simulink model "M1DCSSimulator_M1BcoordinateSystem"  (R2021a)
settings: Solver=VariableStepAuto  StartTime=0.0  StopTime=10.0  RelTol=1e-3
undefined symbols (not defined in the file or in its folder): DiscIntNeverNeededParam
settings Model: Creator=tranka  LastModifiedBy=tranka

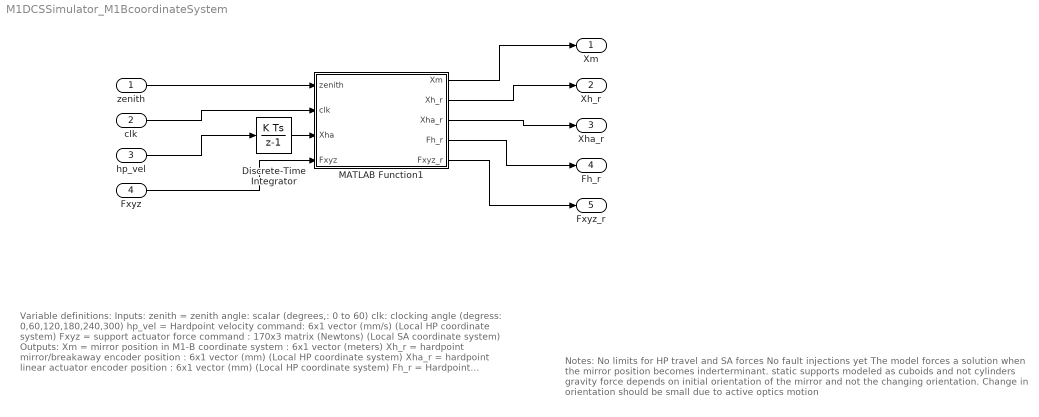
== system M1DCSSimulator_M1BcoordinateSystem ==
  note: Variable definitions:
      |
      | Inputs:
      | zenith = zenith angle: scalar (degrees,: 0 to 60)
      | clk: clocking angle (degress: 0,60,120,180,240,300)
      | hp_vel = Hardpoint velocity command: 6x1 vector (mm/s) (Local HP coordinate system)
      | Fxyz = support actuator force command : 170x3 matrix (Newtons) (Local SA coordinate system)
      |
      | Outputs:
      | Xm = mirror position in M1-B coordinate system : 6x1 vector (meters)
      | Xh_r = hardpoint mirror/breakaway encoder position : 6x1 vector (mm) (Local HP coordinate system)
      | Xha_r = hardpoint linear actuator encoder position : 6x1 vector (mm) (Local HP coordinate system)
      | Fh_r = Hardpoint loadcell readout : 6x1 vector (Newtons) (Local HP coordinate system)
      | FXYZ_r = support actuator force readback : 165x3 matrix (M1B coordinate system. Need to be fixed to local SA coordinate system)
  note: Notes:
      | No limits for HP travel and SA forces
      | No fault injections yet
      | The model forces a solution when the mirror position becomes inderterminant.
      | static supports modeled as cuboids and not cylinders
      | gravity force depends on initial orientation of the mirror and not the changing orientation.
      | Change in orientation should be small due to active optics motion
  zenith : Inport
  clk : Inport  Port=2
  hp_vel : Inport  Port=3
  Fxyz : Inport  Port=4
  Discrete-Time Integrator : DiscreteIntegrator  SampleTime=-1  ICPrevOutput=DiscIntNeverNeededParam  ICPrevScaledInput=DiscIntNeverNeededParam
  MATLAB Function1 : MATLAB Function  TreatAsAtomicUnit=on
  Xm : Outport
  Xh_r : Outport  Port=2
  Xha_r : Outport  Port=3
  Fh_r : Outport  Port=4
  Fxyz_r : Outport  Port=5
  wires:
  Discrete-Time Integrator/1 -> MATLAB Function1/3(Xha)
  zenith/1 -> MATLAB Function1/1(zenith)
  clk/1 -> MATLAB Function1/2(clk)
  hp_vel/1 -> Discrete-Time Integrator/1
  Fxyz/1 -> MATLAB Function1/4(Fxyz)
  MATLAB Function1/1(Xm) -> Xm/1
  MATLAB Function1/2(Xh_r) -> Xh_r/1
  MATLAB Function1/3(Xha_r) -> Xha_r/1
  MATLAB Function1/4(Fh_r) -> Fh_r/1
  MATLAB Function1/5(Fxyz_r) -> Fxyz_r/1

== matlab function M1DCSSimulator_M1BcoordinateSystem/MATLAB Function1 ==
  data: zenith input; clk input; Xm output; Xha input; Fxyz input; Xh_r output; Xha_r output; Fh_r output; Fxyz_r output
function [Xm,Xh_r,Xha_r,Fh_r, Fxyz_r] = mirror(zenith,clk, Xha,Fxyz)
%% fix input coordinates, indexes, units etc
% pass the support actuator to output
% In future implement SA force limits or disable a few actuators.
Fxyz_r = Fxyz;
sign_matrix = [-1    -1    -1
    -1    -1    -1
    -1    -1    -1
    -1    -1    -1
     1     1    -1
     1     1    -1
    -1    -1    -1
    -1    -1    -1
    -1    -1    -1
    -1    -1    -1
    -1    -1    -1
     1     1    -1
    -1    -1    -1
    -1    -1    -1
    -1    -1    -1
    -1    -1    -1
     1     1    -1
     1     1    -1
    -1    -1    -1
    -1    -1    -1
    -1    -1    -1
    -1    -1    -1
     1     1    -1
     1     1    -1
    -1    -1    -1
    -1    -1    -1
    -1    -1    -1
     1     1    -1
     1     1    -1
    -1    -1    -1
    -1    -1    -1
     1     1    -1
     1     1    -1
     1     1    -1
     1     1    -1
     1     1    -1
     1     1    -1
     1     1    -1
     1     1    -1
     1     1    -1
     1     1    -1
     1     1    -1
     1     1    -1
     1     1    -1
     1     1    -1
     1     1    -1
     1     1    -1
     1     1    -1
     1     1    -1
     1     1    -1
     1     1    -1
     1     1    -1
     1     1    -1
     1     1    -1
     1     1    -1
     1     1    -1
     1     1    -1
     1     1    -1
     1     1    -1
     1     1    -1
     1     1    -1
     1     1    -1
     1     1    -1
     1     1    -1
     1     1    -1
     1     1    -1
     1     1    -1
     1     1    -1
     1     1    -1
     1     1    -1
     1     1    -1
     1     1    -1
     1     1    -1
     1     1    -1
     1     1    -1
     1     1    -1
     1     1    -1
     1     1    -1
     1     1    -1
     1     1    -1
     1     1    -1
     1     1    -1
     1     1    -1
     1     1    -1
     1     1    -1
     1     1    -1
     1     1    -1
     1     1    -1
     1     1    -1
     1     1    -1
     1     1    -1
     1     1    -1
     1     1    -1
     1     1    -1
     1     1    -1
     1     1    -1
     1     1    -1
     1     1    -1
     1     1    -1
     1     1    -1
     1     1    -1
     1     1    -1
     1     1    -1
     1     1    -1
     1     1    -1
     1     1    -1
     1     1    -1
     1     1    -1
     1     1    -1
     1     1    -1
     1     1    -1
     1     1    -1
     1     1    -1
     1     1    -1
     1     1    -1
     1     1    -1
     1     1    -1
    -1    -1    -1
    -1    -1    -1
    -1    -1    -1
    -1    -1    -1
    -1    -1    -1
     1     1    -1
    -1    -1    -1
    -1    -1    -1
    -1    -1    -1
    -1    -1    -1
     1     1    -1
     1     1    -1
    -1    -1    -1
    -1    -1    -1
    -1    -1    -1
    -1    -1    -1
     1     1    -1
     1     1    -1
    -1    -1    -1
    -1    -1    -1
    -1    -1    -1
     1     1    -1
     1     1    -1
    -1    -1    -1
    -1    -1    -1
     1     1    -1
     1     1    -1
     1     1    -1
     1     1    -1
     1     1    -1
     1     1    -1
     1     1    -1
     1     1    -1
     1     1    -1
     1     1    -1
     1     1    -1
     1     1    -1
     1     1    -1
     1     1    -1
     1     1    -1
     1     1    -1
     1     1    -1
     1     1    -1
     1     1    -1
     1     1    -1
     1     1    -1
     1     1    -1
     1     1    -1
    -1    -1    -1
    -1    -1    -1
    -1    -1    -1
    -1    -1    -1
    -1    -1    -1];
Fxyz = sign_matrix.*Fxyz;
Fxyz = node_rearangement(Fxyz);
Xha = Xha*1e-3; % millimeter to meter
Xha = -Xha; % HP to M1 B coordinates

%% Constants and transforms
t = 13.5; % tilt of the off axis mirror
% clk = 60; % clocking angle of one of the off axis mirror.

% transforms
% *HP*
% HP2XYZ = [0.38460668	-0.38460668	0.07381907	0.4584258	-0.4584258	-0.07381907;
% 0.30761081	0.30761081	-0.48640517	0.17975252	0.17975252	-0.48640517;
% 0.22921984	0.22921984	0.23032414	0.2293977	0.2293977	0.23032414;
% -0.10285998	-0.10285998	-0.05037601	0.153236	0.153236	-0.05037601;
% -0.11744075	0.11744075	0.14797153	0.03018701	-0.03018701	-0.14797153;
% 0.08255542	-0.08255542	0.08218629	-0.08243407	0.08243407	-0.08218629];

% position M1B to HP coordinate system
XYZ2HP = [-0.45302	0.517744	-0.72575	1.934433	-1.14293	-2.02285;
0.453021	0.517744	-0.72575	1.934433	1.14293	2.02285;
-0.22187	-0.6512	-0.72575	0.02259	2.246733	-2.02285;
-0.67489	0.133456	-0.72575	-1.95702	1.103803	2.02285;
0.67489	0.133456	-0.72575	-1.95702	-1.1038	-2.02285;
0.221869	-0.6512	-0.72575	0.02259	-2.24673	2.02285];

H = -XYZ2HP; %M1B XYZ to M1B HP

% force
HP2XYZ = [-0.45302	0.45302	-0.22187	-0.67489	0.67489	0.22187
0.51774	0.51774	-0.65120	0.13346	0.13346	-0.65120
-0.72575	-0.72575	-0.72575	-0.72575	-0.72575	-0.72575
1.93443	1.93443	0.02259	-1.95702	-1.95702	0.02259
-1.14293	1.14293	2.24673	1.10380	-1.10380	-2.24673
-2.02285	2.02285	-2.02285	2.02285	-2.02285	2.02285];

Th = -HP2XYZ;


% *Equivalent static supports SS*
% Ks_eq = 2.5e5*110; % equivalent static support stiffness
X_ss_gap = [8e-3 8e-3 6.5e-3 8e-3 8e-3 6.5e-3 8e-3 8e-3 6.5e-3]';
% Xm_gap = [8e-3 8e-3 6.5e-3 0 0 0]';

sr1y = 3; sr1x = 0;
sr2x = 3*cosd(210);sr2y = 3*sind(210);
sr3x = 3*cosd(330);sr3y = 3*sind(330);

S2M = [1 0 0 1 0 0 1 0 0;
         0 1 0 0 1 0 0 1 0;
         0 0 1 0 0 1 0 0 1;
         0 0 sr1y 0 0 sr2y 0 0 sr3y;
         0 0 -sr1x 0 0 -sr2x 0 0 -sr3x;
         -sr1y sr1x 0 -sr2y sr2x 0 -sr3y sr3x 0];
% M2S = pinv(S2M);
Ts =     S2M;
ds2dm = [1/3 0 0 1/3 0 0 1/3 0 0;
         0 1/3 0 0 1/3 0 0 1/3 0;
         0 0 1/3 0 0 1/3 0 0 1/3;
         0 0 sr1y 0 0 sr2y 0 0 sr3y;
         0 0 -sr1x 0 0 -sr2x 0 0 -sr3x;
         -sr1y sr1x  0 -sr2y sr2x 0 -sr3y sr3x 0];
S = pinv(ds2dm);
% Ts = ds2dm;

%% persistent variables
persistent Fa_prev  Xm_prev;
% persistent Xha_prev;


if isempty(Fa_prev)
    Fa_prev = zeros(6,1);
end



%% initial down condition

[~, ~, FMg] = decompose_gravity_vector(t,clk,zenith); % decompose gravity vector

if isempty(Xm_prev)
    Fss = Force_M2S(-(FMg+Fa_prev)); % static support reaction force
    Xs = ss_compression_tension(Fss); % static support compression/tension under mirror weight
    Xs = Xs + sign(Xs).*X_ss_gap;
    Xm_prev = Slength2Mlength(Xs); % mirror position 
    Xs0 = sign(Xs).*X_ss_gap;
    Xha = dm2dh(Slength2Mlength(Xs0));
end
if isempty(Xha)
    Xha = dm2dh(Slength2Mlength(Xs0));
end

%% static support stiffness update

Xs = Mlength2Slength(Xm_prev); % mirror position at equivalent static supports
Ks = ss_stiffness(Xs);

%% Support actuator force and moment applied

FMa = ActForces2FM(Fxyz);

%% hardpoint force due to motion of hardpoint actuator only
% during chase
Xh_r = dm2dh(Xm_prev);
[~, Kh, Fhbk] = hp_stiffness(Xh_r,Xha);

% after chase
if (FMg+FMa) < 100 
    Kh = 120e6*eye(6);
    Fhbk = zeros(6,1);
end

%% new mirror position to to support actuator force update
% Xm in M1B
Xm = pinv(Ts*Ks*S + Th*Kh*H)*(FMg + FMa + Ts*Ks*(sign(Xs).*X_ss_gap) + Th*Kh*Xha + Th*Fhbk );


%% hardopint reaction force and mirror encoder update
Xh_r = dm2dh(Xm);
[Fh_r, ~, ~] = hp_stiffness(Xh_r,Xha);

%% update variables for simulation and outputs
Fa_prev = FMa;
Xm_prev = Xm; % in M1B
Xh_r = -Xh_r*1e3; % change it to HP coordinate system and mm
% Fxyz_r = sign_matrix.*Fxyz; % change it to local actuator coordinate system
% Fxyz_r = Fxyz;
Xha_r = -Xha*1e3; % change it to HP coordinate system and mm
